simulink model "db_template_model"  (R2023b)
settings: Solver=VariableStepAuto  StartTime=0.0  StopTime=10.0  RelTol=1e-3
settings Model: Creator=diell  LastModifiedBy=diell
settings RTWCC: GPUComputeCapability=5.0

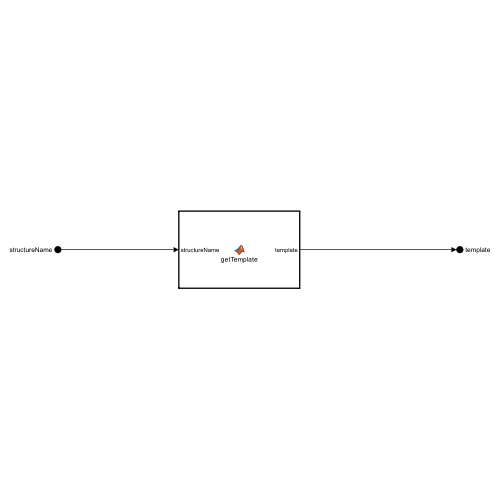
[thumbnail: Simulink's stored preview of the top-level diagram]
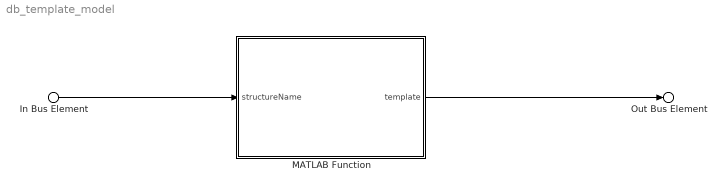
== system db_template_model ==
  In Bus Element : Inport  PortName=structureName
  MATLAB Function : MATLAB Function  TreatAsAtomicUnit=on
  Out Bus Element : Outport  PortName=template
  wires:
  MATLAB Function/1(template) -> Out Bus Element/1
  In Bus Element/1 -> MATLAB Function/1(structureName)

== matlab function db_template_model/MATLAB Function ==
  data: structureName input; template output string
function template = getTemplate(structureName)
    template = db_template(structureName);
end
